simulink model "ProjectStep11"  (R2025b)
settings: Solver=VariableStepAuto  StartTime=0.0  StopTime=10.0  RelTol=1e-3
values from neighbouring files (symbols this model uses):
  A_b = [0 1 0 0; num21_a/Z num22_a/(R*Z) 0 num24_a/(R*r*Z) ; 0 0 0 1; num41_a/Z num42_a/(R*Z) 0 num44_a/(R*Z)]    [Project.m]    (also in Project_Jayce.m = double(vpa(A_b,14)); Project_template.m = [])
  B_b = [0; num2_b/den1_b ; 0; num4_b/den1_b]    [Project.m]    (also in Project_Jayce.m = double(vpa(B_b,14)); Project_template.m = [])
  C_b = [1 0 0 0; 0 1 0 0; 0 0 1 0; 0 0 0 1]    [Project.m]    (also in Project_Jayce.m = eye(size(A_b)); Project_template.m = [])
  D_b = [0; 0; 0; 0]    [Project.m]    (also in Project_Jayce.m = [0;0;0;0]; Project_template.m = [])
  Lgain = place(A_b', C_b', new_poles)'    [Project.m]
  xM0 = [0; 0; 0; 0]    [Project.m]
  xS0 = [0;0;0;0]    [Project.m]
settings Model: Creator=Matthew  LastModifiedBy=Matthew

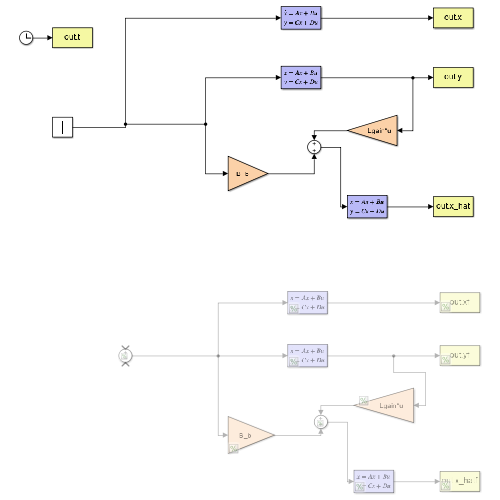
[thumbnail: Simulink's stored preview of the top-level diagram]
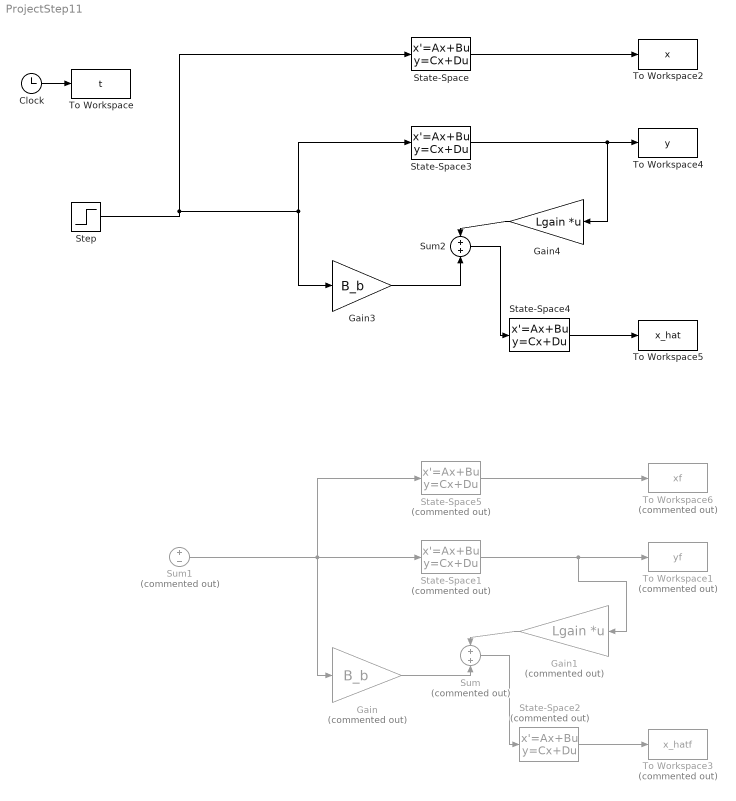
== system ProjectStep11 ==
  Clock : Clock
  Gain : Gain  Commented=on  Gain=B_b
  Gain1 : Gain  Commented=on  Gain=Lgain  Multiplication=Matrix(K*u)
  Gain3 : Gain  Gain=B_b
  Gain4 : Gain  Gain=Lgain  Multiplication=Matrix(K*u)
  State-Space : StateSpace  A=A_b  B=B_b  C=eye(4)  D=[0;0;0;0]  InitialCondition=xS0
  State-Space1 : StateSpace  Commented=on  A=A_b  B=B_b  C=C_b  D=D_b  InitialCondition=xS0
  State-Space2 : StateSpace  Commented=on  A=A_b-Lgain*C_b  B=eye(4)  C=eye(4)  D=zeros(4,4)  InitialCondition=xM0
  State-Space3 : StateSpace  A=A_b  B=B_b  C=C_b  D=D_b  InitialCondition=xS0
  State-Space4 : StateSpace  A=A_b-Lgain*C_b  B=eye(4)  C=eye(4)  D=zeros(4,4)  InitialCondition=xM0
  State-Space5 : StateSpace  Commented=on  A=A_b  B=B_b  C=eye(size(A_b))  D=zeros(size(C_b,1),size(B_b,2))  InitialCondition=xS0
  Step : Step  SampleTime=0
  Sum : Sum  Commented=on
  Sum1 : Sum  Commented=on  Inputs=+|-
  Sum2 : Sum
  To Workspace : ToWorkspace  VariableName=t  SampleTime=-1
  To Workspace1 : ToWorkspace  Commented=on  VariableName=yf  SampleTime=-1
  To Workspace2 : ToWorkspace  VariableName=x  SampleTime=-1
  To Workspace3 : ToWorkspace  Commented=on  VariableName=x_hatf  SampleTime=-1
  To Workspace4 : ToWorkspace  VariableName=y  SampleTime=-1
  To Workspace5 : ToWorkspace  VariableName=x_hat  SampleTime=-1
  To Workspace6 : ToWorkspace  Commented=on  VariableName=xf  SampleTime=-1
  wires:
  State-Space3/1 -> Gain4/1, To Workspace4/1
  State-Space4/1 -> To Workspace5/1
  State-Space1/1 -> To Workspace1/1, Gain1/1
  Gain3/1 -> Sum2/2
  Sum/1 -> State-Space2/1
  State-Space2/1 -> To Workspace3/1
  Sum1/1 -> State-Space5/1, Gain/1, State-Space1/1
  Gain4/1 -> Sum2/1
  Gain1/1 -> Sum/1
  Clock/1 -> To Workspace/1
  State-Space5/1 -> To Workspace6/1
  Sum2/1 -> State-Space4/1
  State-Space/1 -> To Workspace2/1
  Step/1 -> State-Space/1, State-Space3/1, Gain3/1
  Gain/1 -> Sum/2
